simulink model "solar_panel_test_simple"  (R2016b)
settings: Solver=VariableStepAuto  StartTime=0.0  StopTime=1000  RelTol=1e-3
libraries: aerolibtransform2 x1, dynamics_lib x1, solar_panel_power_lib x1
settings Model: Creator=taylorreynolds  LastModifiedBy=taylorreynolds

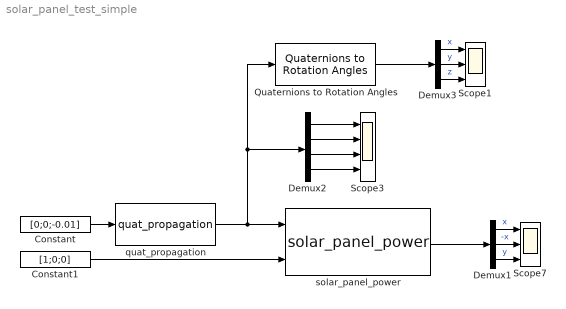
== system solar_panel_test_simple ==
  Constant : Constant  Value=[0;0;-0.01]
  Constant1 : Constant  Value=[1;0;0]
  Demux1 : Demux  Outputs=3
  Demux2 : Demux
  Demux3 : Demux  Outputs=3
  Quaternions to Rotation Angles : aerolibtransform2/Quaternions to Rotation Angles  rotationOrder=XYZ
  Scope1 : Scope  NumInputPorts=3
  Scope3 : Scope  NumInputPorts=4
  Scope7 : Scope  NumInputPorts=3
  quat_propagation : dynamics_lib/Dynamics/quat_propagation
  solar_panel_power : solar_panel_power_lib/solar_panel_power
  wires:
  Constant/1 -> quat_propagation/1
  quat_propagation/1 -> Quaternions to Rotation Angles/1, Demux2/1, solar_panel_power/1
  Constant1/1 -> solar_panel_power/2
  solar_panel_power/1 -> Demux1/1
  Demux1/2 -> Scope7/2  "-x"
  Demux1/1 -> Scope7/1  "x"
  Demux1/3 -> Scope7/3  "y"
  Demux2/3 -> Scope3/3
  Demux2/4 -> Scope3/4
  Demux2/2 -> Scope3/2
  Demux2/1 -> Scope3/1
  Quaternions to Rotation Angles/1 -> Demux3/1
  Demux3/2 -> Scope1/2  "y"
  Demux3/1 -> Scope1/1  "x"
  Demux3/3 -> Scope1/3  "z"
